simulink model "Demo_CarRealTime2D_cs"  (R2014b)
settings: Solver=ode5  SolverMode=SingleTasking  StartTime=0.0  StopTime=inf  FixedStep=1/1000  RelTol=1e-3
PreLoadFcn:
  | mbxruntime.callbacks.PreLoadFcn(bdroot);
  | check_NUTS_defined;
  | assignin('base',['model_closed_' bdroot],false);
  | addpath('../includes_AEBS');
PostLoadFcn:
  | mbxruntime.callbacks.PostLoadFcn(bdroot);
InitFcn:
  | mbxruntime.callbacks.InitFcn(bdroot);
StartFcn:
  | mbxruntime.callbacks.StartFcn(bdroot);
StopFcn:
  | mbxruntime.callbacks.StopFcn(bdroot);;
  | 
model workspace: external: MAT-File .\Demo_CarRealTime2D_cs_hws.mat (data not in the file)
undefined symbols (not defined in the file or in its folder): Driver_Demands, mbxruntime, tabledata, vicrt_initcallback, vicrt_initmexcallback, vicrt_simulationmanager, warningInitialVelocity, x0
undefined symbols (not defined in the file): Demo_CarRealTime2D_cs_007c1c37f387f47f, Demo_CarRealTime2D_cs_085a64a83ba38cec, Demo_CarRealTime2D_cs_0a7f542d3fc7ab9f, Demo_CarRealTime2D_cs_0d7c72cfaa56dff7, Demo_CarRealTime2D_cs_0de07b35068e3828, Demo_CarRealTime2D_cs_17f4d381375cce95, Demo_CarRealTime2D_cs_1db40a09b08215a9, Demo_CarRealTime2D_cs_2bfa3850c176687b, Demo_CarRealTime2D_cs_35a34f1ba6ce4a22, Demo_CarRealTime2D_cs_378cc77e08d643fb, Demo_CarRealTime2D_cs_409b5c3befba0000, Demo_CarRealTime2D_cs_42628ca5bb62d2f3, Demo_CarRealTime2D_cs_56554a2db408a7f8, Demo_CarRealTime2D_cs_59527455249d7429, Demo_CarRealTime2D_cs_5983ee1b8112afac, Demo_CarRealTime2D_cs_5b5ebcf3ed7bf8e6, Demo_CarRealTime2D_cs_63cbe7fbe16cd5d9, Demo_CarRealTime2D_cs_6e17b9adbf989abf, Demo_CarRealTime2D_cs_6f662a34e5d9a196, Demo_CarRealTime2D_cs_75c4ee8892821e19, Demo_CarRealTime2D_cs_7c64486355814be2, Demo_CarRealTime2D_cs_849809550a2230ef, Demo_CarRealTime2D_cs_87f899bcbe16d8f5, Demo_CarRealTime2D_cs_8e7b50dac25b68a2, Demo_CarRealTime2D_cs_94938e5260f139b3, Demo_CarRealTime2D_cs_983acc940698d1d1, Demo_CarRealTime2D_cs_9d554c72797f76fd, Demo_CarRealTime2D_cs_9d747ee2f15c057f, Demo_CarRealTime2D_cs_ad62a2084d31e898, Demo_CarRealTime2D_cs_b56c8c5f000d30f0, Demo_CarRealTime2D_cs_b95f1b7356e926cc, Demo_CarRealTime2D_cs_BMW_X5_1_Path_pathUniqueID, Demo_CarRealTime2D_cs_BMW_Z3_2_Dynamics_Empty_STATE_BMW_Z3_2_x0, Demo_CarRealTime2D_cs_BMW_Z3_2_Dynamics_Empty_STATE_BMW_Z3_2_y0, Demo_CarRealTime2D_cs_BMW_Z3_2_Dynamics_Empty_STATE_BMW_Z3_2_z0, Demo_CarRealTime2D_cs_BMW_Z3_Path_pathUniqueID, Demo_CarRealTime2D_cs_BMW_Z3_SpeedProfile_speedProfileUniqueID, Demo_CarRealTime2D_cs_c8847ab2e5633224, Demo_CarRealTime2D_cs_c9a0d701286b93fb, Demo_CarRealTime2D_cs_ce758cae7dd1b283, Demo_CarRealTime2D_cs_CrossingPedestrian_Path_pathUniqueID, Demo_CarRealTime2D_cs_CuttingInVehicle_Path_pathUniqueID, Demo_CarRealTime2D_cs_d901ab1c1d2e40bc, Demo_CarRealTime2D_cs_dff70430e5a00a86, Demo_CarRealTime2D_cs_ef038a4f619ad32e, Demo_CarRealTime2D_cs_Female_OverweightAni_1_Path_pathUniqueID, Demo_CarRealTime2D_cs_Ford_Fiesta_1_Path_pathUniqueID, Demo_CarRealTime2D_cs_Ford_FocusWagon_Path_pathUniqueID, Demo_CarRealTime2D_cs_Sphere_1_Dynamics_Empty_STATE_Sphere_1_x0, Demo_CarRealTime2D_cs_Sphere_1_Dynamics_Empty_STATE_Sphere_1_y0, Demo_CarRealTime2D_cs_Sphere_1_Dynamics_Empty_STATE_Sphere_1_z0, WheelL0, WheelL1, WheelR0, WheelR1
libraries: PreScanSimulinkLibrary x15, simulink x15, simulink_extras x15, PreScanUsefulBlocks x2, dspsigops x1
(part 16 of 17)

== system Demo_CarRealTime2D_cs/HostVehicle/PathFollower_Preview_1/LateralController/SteeringWheelAngle/FirstOrderDynamics ==
  In : Inport
  TimeConstant[s] : Inport  Port=2
  Reset : Inport  Port=3
  x0 : Inport  Port=4
  1|TimeConstant : Product  Inputs=*/  SaturateOnIntegerOverflow=on  InputSameDT=on  OutDataTypeStr=Inherit: Same as first input
  Discrete-Time Integrator : DiscreteIntegrator  ExternalReset=rising  InitialConditionSource=external  InitialCondition=x0  SampleTime=CSSampleTime
  IC : InitialCondition  Value=0
  Saturation : Saturate  UpperLimit=1e300  LowerLimit=0.001
  Sum : Sum  Inputs=-+|  SaturateOnIntegerOverflow=on  InputSameDT=on  OutDataTypeStr=Inherit: Same as first input
  Out : Outport
  wires:
  IC/1 -> Discrete-Time Integrator/3
  In/1 -> Sum/2
  x0/1 -> IC/1
  Reset/1 -> Discrete-Time Integrator/2
  1|TimeConstant/1 -> Discrete-Time Integrator/1
  Sum/1 -> 1|TimeConstant/1
  Saturation/1 -> 1|TimeConstant/2
  TimeConstant[s]/1 -> Saturation/1
  Discrete-Time Integrator/1 -> Out/1, Sum/1

== system Demo_CarRealTime2D_cs/HostVehicle/PathFollower_Preview_1/LateralController/SteeringWheelAngle/Sat_Total ==
  In : Inport
  Sat_Limit : Inport  Port=2
  Gain1 : Gain  Gain=-1  SaturateOnIntegerOverflow=on  OutDataTypeStr=Inherit: Same as input  ParamDataTypeStr=Inherit: Same as input
  RelOp_UL : RelationalOperator
  RelOp_UL1 : RelationalOperator  Operator=<=
  Sum : Sum  Inputs=++|  SaturateOnIntegerOverflow=on
  Switch : Switch  Threshold=0.5  SaturateOnIntegerOverflow=on
  Switch1 : Switch  Threshold=0.5  SaturateOnIntegerOverflow=on
  Sat_Total : Outport
  Sat_Info : Outport  Port=2
  wires:
  Sat_Limit/1 -> Gain1/1, Switch/1, RelOp_UL/2
  RelOp_UL/1 -> Switch/2, Sum/2
  Switch/1 -> RelOp_UL1/1, Switch1/3
  Gain1/1 -> RelOp_UL1/2, Switch1/1
  RelOp_UL1/1 -> Switch1/2, Sum/1
  In/1 -> Switch/3, RelOp_UL/1
  Switch1/1 -> Sat_Total/1
  Sum/1 -> Sat_Info/1

== system Demo_CarRealTime2D_cs/HostVehicle/PathFollower_Preview_1/LongitudinalController/If Desired Velocity ~= 0/PID_AWU ==
  e : Inport
  Derivative Gain : Gain  Gain=D  SaturateOnIntegerOverflow=on  OutDataTypeStr=Inherit: Same as input  ParamDataTypeStr=Inherit: Same as input
  Discrete-Time Integrator : DiscreteIntegrator  gainval=1  SampleTime=CSSampleTime  UpperSaturationLimit=100  LowerSaturationLimit=-100
  Filter : DiscreteIntegrator  gainval=1  SampleTime=CSSampleTime
  Integral Gain : Gain  Gain=I  SaturateOnIntegerOverflow=on  OutDataTypeStr=Inherit: Same as input  ParamDataTypeStr=Inherit: Same as input
  Integral Gain1 : Gain  Gain=LongCtrl_AWU  SaturateOnIntegerOverflow=on  OutDataTypeStr=Inherit: Same as input  ParamDataTypeStr=Inherit: Same as input
  Proportional Gain : Gain  Gain=P  SaturateOnIntegerOverflow=on  OutDataTypeStr=Inherit: Same as input  ParamDataTypeStr=Inherit: Same as input
  Saturation : Saturate  UpperLimit=100  LowerLimit=-100
  Sum : Sum  Inputs=+++  SaturateOnIntegerOverflow=on  InputSameDT=on  OutDataTypeStr=Inherit: Same as first input
  Sum1 : Sum  Inputs=|+-  SaturateOnIntegerOverflow=on  InputSameDT=on  OutDataTypeStr=Inherit: Same as first input
  Sum2 : Sum  Inputs=|++  SaturateOnIntegerOverflow=on  InputSameDT=on  OutDataTypeStr=Inherit: Same as first input
  Sum3 : Sum  Inputs=-+|  SaturateOnIntegerOverflow=on  InputSameDT=on  OutDataTypeStr=Inherit: Same as first input
  u : Outport  InitialOutput=0
  wires:
  Integral Gain1/1 -> Sum2/2
  Sum3/1 -> Integral Gain1/1
  Saturation/1 -> Sum3/2, u/1
  Sum2/1 -> Discrete-Time Integrator/1
  Sum1/1 -> Sum/3, Filter/1
  Filter/1 -> Sum1/2
  Derivative Gain/1 -> Sum1/1
  Sum/1 -> Sum3/1, Saturation/1
  e/1 -> Integral Gain/1, Proportional Gain/1, Derivative Gain/1
  Discrete-Time Integrator/1 -> Sum/2
  Proportional Gain/1 -> Sum/1
  Integral Gain/1 -> Sum2/1

== system Demo_CarRealTime2D_cs/HostVehicle/Vehicles Synchronization/Evaluate_Event_To_Trigger_CuttingVehicle/Evaluate Experiment Conditions /Compute Components ==
  R [m] : Inport
  Th [deg] : Inport  Port=2
  Degrees to Radians : simulink_extras/Transformations/Degrees to Radians
  Product1 : Product  RndMeth=Zero
  Product8 : Product  RndMeth=Zero
  Trigonometric Function1 : Trigonometry  Operator=cos
  Trigonometric Function3 : Trigonometry
  delta_x [m] : Outport
  delta_y [m] : Outport  Port=2
  wires:
  Th [deg]/1 -> Degrees to Radians/1
  Product1/1 -> delta_y [m]/1
  Trigonometric Function3/1 -> Product1/2
  Product8/1 -> delta_x [m]/1
  Trigonometric Function1/1 -> Product8/2
  R [m]/1 -> Product8/1, Product1/1
  Degrees to Radians/1 -> Trigonometric Function1/1, Trigonometric Function3/1

== system Demo_CarRealTime2D_cs/HostVehicle/Vehicles Synchronization/Evaluate_Event_To_Trigger_CuttingVehicle/Evaluate Experiment Conditions /Compute Relative Longitudional Velocity ==
  V_Det [m/s] : Inport
  HV_V [m/s] : Inport  Port=2
  Abs : Abs
  Sum : Sum  Inputs=|+-
  delta_V [m/s] : Outport
  wires:
  Abs/1 -> delta_V [m/s]/1
  Sum/1 -> Abs/1
  HV_V [m/s]/1 -> Sum/2
  V_Det [m/s]/1 -> Sum/1

== system Demo_CarRealTime2D_cs/HostVehicle/Vehicles Synchronization/Evaluate_Event_To_Trigger_CuttingVehicle/Evaluate Experiment Conditions /Compute Vehcile Position Bend Road ==
  R [m] : Inport
  Th [deg] : Inport  Port=2
  delta_x [m] : Inport  Port=3
  HV_V [m/s] : Inport  Port=4
  HV_YawRate [deg/s] : Inport  Port=5
  Action Port : ActionPort
  Compare To Constant : simulink/Logic and Bit Operations/Compare To Constant  relop=<  const=0  OutDataTypeStr=boolean
  Compare To Constant1 : simulink/Logic and Bit Operations/Compare To Constant  relop=>  const=0  OutDataTypeStr=boolean
  Compare To Constant2 : simulink/Logic and Bit Operations/Compare To Constant  relop=>  const=0  OutDataTypeStr=boolean
  Compare To Constant3 : simulink/Logic and Bit Operations/Compare To Constant  relop=<  const=0  OutDataTypeStr=boolean
  Dead Zone : DeadZone  LowerValue=-0.1  UpperValue=0.1  SaturateOnIntegerOverflow=on
  Dead Zone1 : DeadZone  LowerValue=-0.1  UpperValue=0.1  SaturateOnIntegerOverflow=on
  Scope : Scope
      settings: YMin=-2.75  YMax=0.25  SaveName=ScopeData2
  Sign : Signum
  Sign1 : Signum
  TV on same lane : Subsystem
  "TV_front " : Outport
  TV_rear : Outport  Port=2
  TV_left : Outport  Port=3
  TV_right : Outport  Port=4
  y_pos_traj : Outport  Port=5
  wires:
  Dead Zone1/1 -> Sign1/1
  Dead Zone/1 -> Sign/1
  Compare To Constant1/1 -> TV_right/1
  HV_YawRate [deg/s]/1 -> TV on same lane/4(HV_Yaw_rate_[deg/s])
  HV_V [m/s]/1 -> TV on same lane/3(HV_Velocity [m/s])
  Th [deg]/1 -> TV on same lane/2(Th_Sensor deg])
  R [m]/1 -> TV on same lane/1(Range_Sensor [m])
  delta_x [m]/1 -> Dead Zone/1
  Sign/1 -> Compare To Constant/1, Compare To Constant2/1
  Compare To Constant/1 -> TV_rear/1
  TV on same lane/1(y_pos_traj) -> y_pos_traj/1, Scope/1, Dead Zone1/1
  Sign1/1 -> Compare To Constant1/1, Compare To Constant3/1
  Compare To Constant2/1 -> "TV_front "/1
  Compare To Constant3/1 -> TV_left/1

== system Demo_CarRealTime2D_cs/HostVehicle/Vehicles Synchronization/Evaluate_Event_To_Trigger_CuttingVehicle/Evaluate Experiment Conditions /Compute Vehcile Position Sraight Road ==
  delta_x [m] : Inport
  delta_y [m] : Inport  Port=2
  Action Port : ActionPort
  Compare To Constant : simulink/Logic and Bit Operations/Compare To Constant  relop=<  const=0  OutDataTypeStr=boolean
  Compare To Constant1 : simulink/Logic and Bit Operations/Compare To Constant  relop=>  const=0  OutDataTypeStr=boolean
  Compare To Constant2 : simulink/Logic and Bit Operations/Compare To Constant  relop=>  const=0  OutDataTypeStr=boolean
  Compare To Constant3 : simulink/Logic and Bit Operations/Compare To Constant  relop=<  const=0  OutDataTypeStr=boolean
  Dead Zone : DeadZone  LowerValue=-0.1  UpperValue=0.1  SaturateOnIntegerOverflow=on
  Dead Zone1 : DeadZone  LowerValue=-0.1  UpperValue=0.1  SaturateOnIntegerOverflow=on
  Sign : Signum
  Sign1 : Signum
  "TV_front " : Outport
  TV_rear : Outport  Port=2
  TV_left : Outport  Port=3
  TV_right : Outport  Port=4
  wires:
  Dead Zone1/1 -> Sign1/1
  Dead Zone/1 -> Sign/1
  Compare To Constant3/1 -> TV_left/1
  Compare To Constant2/1 -> "TV_front "/1
  Compare To Constant1/1 -> TV_right/1
  Sign1/1 -> Compare To Constant3/1, Compare To Constant1/1
  delta_y [m]/1 -> Dead Zone1/1
  Compare To Constant/1 -> TV_rear/1
  Sign/1 -> Compare To Constant2/1, Compare To Constant/1
  delta_x [m]/1 -> Dead Zone/1

== system Demo_CarRealTime2D_cs/HostVehicle/Vehicles Synchronization/Evaluate_Event_To_Trigger_CuttingVehicle/Evaluate Experiment Conditions /Straight or Curved Road Scenario ==
  note: === Switching block ===
      |
      |  - determines if the HV is moving on a straight road or on a bend raod,
      |  - based on the actual value of the yaw rate of the HV.
  EGO_Yaw_rate_[deg/s] : Inport
  1deg_per_s : Constant
  Abs : Abs
  Bend_Road [2] : Constant  Value=2
  Relational Operator : RelationalOperator  Operator=<  OutDataTypeStr=boolean
  Straight_Road [1] : Constant
  Switch : Switch  Criteria=u2 ~= 0  Threshold=0.5
  Sraight[1] / Bend[2] : Outport
  wires:
  Bend_Road [2]/1 -> Switch/3
  Straight_Road [1]/1 -> Switch/1
  Abs/1 -> Relational Operator/1
  Switch/1 -> Sraight[1] / Bend[2]/1
  Relational Operator/1 -> Switch/2
  1deg_per_s/1 -> Relational Operator/2
  EGO_Yaw_rate_[deg/s]/1 -> Abs/1

== system Demo_CarRealTime2D_cs/CuttingInVehicle/Trajectories1/Traj2State1/Traj2State2/Traj2MuxState_Ext/demux ==
  traj : Inport
  Demux : Demux  Outputs=18
  x : Outport
  y : Outport  Port=2
  z : Outport  Port=3
  velx : Outport  Port=4
  vely : Outport  Port=5
  velz : Outport  Port=6
  R : Outport  Port=7
  P : Outport  Port=8
  Y : Outport  Port=9
  velR : Outport  Port=10
  velP : Outport  Port=11
  velY : Outport  Port=12
  accx : Outport  Port=13
  accy : Outport  Port=14
  accz : Outport  Port=15
  accR : Outport  Port=16
  accP : Outport  Port=17
  accY : Outport  Port=18
  wires:
  Demux/1 -> x/1
  Demux/2 -> y/1
  Demux/3 -> z/1
  Demux/4 -> R/1
  traj/1 -> Demux/1
  Demux/5 -> P/1
  Demux/6 -> Y/1
  Demux/7 -> velx/1
  Demux/8 -> vely/1
  Demux/9 -> velz/1
  Demux/10 -> velR/1
  Demux/11 -> velP/1
  Demux/12 -> velY/1
  Demux/13 -> accx/1
  Demux/14 -> accy/1
  Demux/15 -> accz/1
  Demux/16 -> accR/1
  Demux/17 -> accP/1
  Demux/18 -> accY/1

== system Demo_CarRealTime2D_cs/HostVehicle/Dynamics_UserSpecified/VI-CarRealTime/Input_Bus/Inputs/Aerodynamic ==
  BCAerodynamic : BusCreator  Inputs=12
  fx_center_def_val : Constant  Value=0
  fx_front_def_val : Constant  Value=0
  fx_rear_def_val : Constant  Value=0
  fy_center_def_val : Constant  Value=0
  fy_front_def_val : Constant  Value=0
  fy_rear_def_val : Constant  Value=0
  fz_center_def_val : Constant  Value=0
  fz_front_def_val : Constant  Value=0
  fz_rear_def_val : Constant  Value=0
  mx_def_val : Constant  Value=0
  my_def_val : Constant  Value=0
  mz_def_val : Constant  Value=0
  Aerodynamic : Outport
  wires:
  mz_def_val/1 -> BCAerodynamic/12  "mz"
  my_def_val/1 -> BCAerodynamic/11  "my"
  mx_def_val/1 -> BCAerodynamic/10  "mx"
  fz_center_def_val/1 -> BCAerodynamic/9  "fz_center"
  fy_center_def_val/1 -> BCAerodynamic/8  "fy_center"
  fx_center_def_val/1 -> BCAerodynamic/7  "fx_center"
  fz_rear_def_val/1 -> BCAerodynamic/6  "fz_rear"
  fy_rear_def_val/1 -> BCAerodynamic/5  "fy_rear"
  fx_rear_def_val/1 -> BCAerodynamic/4  "fx_rear"
  fz_front_def_val/1 -> BCAerodynamic/3  "fz_front"
  fy_front_def_val/1 -> BCAerodynamic/2  "fy_front"
  fx_front_def_val/1 -> BCAerodynamic/1  "fx_front"
  BCAerodynamic/1 -> Aerodynamic/1  "Aerodynamic"

== system Demo_CarRealTime2D_cs/HostVehicle/Dynamics_UserSpecified/VI-CarRealTime/Input_Bus/Inputs/Antiroll_Bar ==
  BCAntiroll_Bar : BusCreator  Inputs=2
  activity_flag : Subsystem
  force : Subsystem
  Antiroll_Bar : Outport
  wires:
  force/1(force) -> BCAntiroll_Bar/2  "force"
  activity_flag/1(activity_flag) -> BCAntiroll_Bar/1  "activity_flag"
  BCAntiroll_Bar/1 -> Antiroll_Bar/1  "Antiroll_Bar"

== system Demo_CarRealTime2D_cs/HostVehicle/Dynamics_UserSpecified/VI-CarRealTime/Input_Bus/Inputs/Auxiliary_vertical ==
  BCAuxiliary_vertical : BusCreator  Inputs=2
  activity_flag : Subsystem
  force : Subsystem
  Auxiliary_vertical : Outport
  wires:
  activity_flag/1(activity_flag) -> BCAuxiliary_vertical/2  "activity_flag"
  force/1(force) -> BCAuxiliary_vertical/1  "force"
  BCAuxiliary_vertical/1 -> Auxiliary_vertical/1  "Auxiliary_vertical"

== system Demo_CarRealTime2D_cs/HostVehicle/Dynamics_UserSpecified/VI-CarRealTime/Input_Bus/Inputs/Brake_System ==
  BCBrake_System : BusCreator  Inputs=5
  brk_mmag_sign : Subsystem
  brk_mmag_unsign : Subsystem
  brk_mu : Subsystem
  brk_pres : Subsystem
  brk_pres_gain : Subsystem
  Brake_System : Outport
  wires:
  brk_mu/1(brk_mu) -> BCBrake_System/5  "brk_mu"
  brk_pres_gain/1(brk_pres_gain) -> BCBrake_System/4  "brk_pres_gain"
  brk_pres/1(brk_pres) -> BCBrake_System/3  "brk_pres"
  brk_mmag_unsign/1(brk_mmag_unsign) -> BCBrake_System/2  "brk_mmag_unsign"
  brk_mmag_sign/1(brk_mmag_sign) -> BCBrake_System/1  "brk_mmag_sign"
  BCBrake_System/1 -> Brake_System/1  "Brake_System"

== system Demo_CarRealTime2D_cs/HostVehicle/Dynamics_UserSpecified/VI-CarRealTime/Input_Bus/Inputs/Brake_System_General ==
  BCBrake_System_General : BusCreator  Inputs=2
  brk_bias_front_def_val : Constant  Value=0
  brk_mast_cyl_pres_def_val : Constant  Value=0
  Brake_System_General : Outport
  wires:
  brk_bias_front_def_val/1 -> BCBrake_System_General/2  "brk_bias_front"
  brk_mast_cyl_pres_def_val/1 -> BCBrake_System_General/1  "brk_mast_cyl_pres"
  BCBrake_System_General/1 -> Brake_System_General/1  "Brake_System_General"

== system Demo_CarRealTime2D_cs/HostVehicle/Dynamics_UserSpecified/VI-CarRealTime/Input_Bus/Inputs/Clutch ==
  BCClutch : BusCreator  Inputs=2
  clutch_slip_angle_def_val : Constant  Value=0
  clutch_trq_def_val : Constant  Value=0
  Clutch : Outport
  wires:
  clutch_slip_angle_def_val/1 -> BCClutch/2  "clutch_slip_angle"
  clutch_trq_def_val/1 -> BCClutch/1  "clutch_trq"
  BCClutch/1 -> Clutch/1  "Clutch"

== system Demo_CarRealTime2D_cs/HostVehicle/Dynamics_UserSpecified/VI-CarRealTime/Input_Bus/Inputs/Driver_Demands ==
  BCDriver_Demands : BusCreator  Inputs=12
  brake_def_val : Constant  Value=0
  clutch_def_val : Constant  Value=0
  gear_def_val : Constant  Value=0
  rack_displacement_def_val : Constant  Value=0
  str_swa_def_val : Constant  Value=0
  throttle_def_val : Constant  Value=0
  user_input_braking_def_val : Constant  Value=0
  user_input_clutch_def_val : Constant  Value=0
  user_input_gear_def_val : Constant  Value=0
  user_input_steering_def_val : Constant  Value=0
  user_input_throttle_def_val : Constant  Value=0
  user_maneuver_ID_def_val : Constant  Value=0
  Driver_Demands : Outport
  wires:
  user_input_clutch_def_val/1 -> BCDriver_Demands/12  "user_input_clutch"
  user_input_gear_def_val/1 -> BCDriver_Demands/11  "user_input_gear"
  user_input_braking_def_val/1 -> BCDriver_Demands/10  "user_input_braking"
  user_input_throttle_def_val/1 -> BCDriver_Demands/9  "user_input_throttle"
  user_input_steering_def_val/1 -> BCDriver_Demands/8  "user_input_steering"
  user_maneuver_ID_def_val/1 -> BCDriver_Demands/7  "user_maneuver_ID"
  brake_def_val/1 -> BCDriver_Demands/6  "brake"
  clutch_def_val/1 -> BCDriver_Demands/5  "clutch"
  gear_def_val/1 -> BCDriver_Demands/4  "gear"
  throttle_def_val/1 -> BCDriver_Demands/3  "throttle"
  rack_displacement_def_val/1 -> BCDriver_Demands/2  "rack_displacement"
  str_swa_def_val/1 -> BCDriver_Demands/1  "str_swa"
  BCDriver_Demands/1 -> Driver_Demands/1  "Driver_Demands"

== system Demo_CarRealTime2D_cs/HostVehicle/Dynamics_UserSpecified/VI-CarRealTime/Input_Bus/Inputs/Engine ==
  BCEngine : BusCreator  Inputs=5
  engine_max_trq_def_val : Constant  Value=0
  engine_min_trq_def_val : Constant  Value=0
  engine_omega_def_val : Constant  Value=0
  engine_trq_def_val : Constant  Value=0
  non_termic_engine_trq_def_val : Constant  Value=0
  Engine : Outport
  wires:
  non_termic_engine_trq_def_val/1 -> BCEngine/5  "non_termic_engine_trq"
  engine_trq_def_val/1 -> BCEngine/4  "engine_trq"
  engine_min_trq_def_val/1 -> BCEngine/3  "engine_min_trq"
  engine_max_trq_def_val/1 -> BCEngine/2  "engine_max_trq"
  engine_omega_def_val/1 -> BCEngine/1  "engine_omega"
  BCEngine/1 -> Engine/1  "Engine"

== system Demo_CarRealTime2D_cs/HostVehicle/Dynamics_UserSpecified/VI-CarRealTime/Input_Bus/Inputs/Ext_Body ==
  BCExt_Body : BusCreator  Inputs=2
  force : Subsystem
  moment : Subsystem
  Ext_Body : Outport
  wires:
  moment/1(moment) -> BCExt_Body/2  "moment"
  force/1(force) -> BCExt_Body/1  "force"
  BCExt_Body/1 -> Ext_Body/1  "Ext_Body"

== system Demo_CarRealTime2D_cs/HostVehicle/Dynamics_UserSpecified/VI-CarRealTime/Input_Bus/Inputs/Ext_Ground ==
  BCExt_Ground : BusCreator  Inputs=2
  force : Subsystem
  moment : Subsystem
  Ext_Ground : Outport
  wires:
  moment/1(moment) -> BCExt_Ground/2  "moment"
  force/1(force) -> BCExt_Ground/1  "force"
  BCExt_Ground/1 -> Ext_Ground/1  "Ext_Ground"

== system Demo_CarRealTime2D_cs/HostVehicle/Dynamics_UserSpecified/VI-CarRealTime/Input_Bus/Inputs/Ext_Tracking ==
  BCExt_Tracking : BusCreator  Inputs=2
  force : Subsystem
  moment : Subsystem
  Ext_Tracking : Outport
  wires:
  moment/1(moment) -> BCExt_Tracking/2  "moment"
  force/1(force) -> BCExt_Tracking/1  "force"
  BCExt_Tracking/1 -> Ext_Tracking/1  "Ext_Tracking"

== system Demo_CarRealTime2D_cs/HostVehicle/Dynamics_UserSpecified/VI-CarRealTime/Input_Bus/Inputs/Friction ==
  BCFriction : BusCreator  Inputs=1
  tire_mu : Subsystem
  Friction : Outport
  wires:
  tire_mu/1(tire_mu) -> BCFriction/1  "tire_mu"
  BCFriction/1 -> Friction/1  "Friction"

== system Demo_CarRealTime2D_cs/HostVehicle/Dynamics_UserSpecified/VI-CarRealTime/Input_Bus/Inputs/GearBox ==
  BCGearBox : BusCreator  Inputs=1
  transmission_ratio_def_val : Constant  Value=0
  GearBox : Outport
  wires:
  transmission_ratio_def_val/1 -> BCGearBox/1  "transmission_ratio"
  BCGearBox/1 -> GearBox/1  "GearBox"

== system Demo_CarRealTime2D_cs/HostVehicle/Dynamics_UserSpecified/VI-CarRealTime/Input_Bus/Inputs/Hook ==
  BCHook : BusCreator  Inputs=6
  Fx : Subsystem
  Fy : Subsystem
  Fz : Subsystem
  Mx : Subsystem
  My : Subsystem
  Mz : Subsystem
  Hook : Outport
  wires:
  Mz/1(Mz) -> BCHook/6  "Mz"
  My/1(My) -> BCHook/5  "My"
  Mx/1(Mx) -> BCHook/4  "Mx"
  Fz/1(Fz) -> BCHook/3  "Fz"
  Fy/1(Fy) -> BCHook/2  "Fy"
  Fx/1(Fx) -> BCHook/1  "Fx"
  BCHook/1 -> Hook/1  "Hook"

== system Demo_CarRealTime2D_cs/HostVehicle/Dynamics_UserSpecified/VI-CarRealTime/Input_Bus/Inputs/Irregularity ==
  BCIrregularity : BusCreator  Inputs=1
  road : Subsystem
  Irregularity : Outport
  wires:
  road/1(road) -> BCIrregularity/1  "road"
  BCIrregularity/1 -> Irregularity/1  "Irregularity"

== system Demo_CarRealTime2D_cs/HostVehicle/Dynamics_UserSpecified/VI-CarRealTime/Input_Bus/Inputs/Main_Bumpstop ==
  BCMain_Bumpstop : BusCreator  Inputs=2
  activity_flag : Subsystem
  force : Subsystem
  Main_Bumpstop : Outport
  wires:
  activity_flag/1(activity_flag) -> BCMain_Bumpstop/2  "activity_flag"
  force/1(force) -> BCMain_Bumpstop/1  "force"
  BCMain_Bumpstop/1 -> Main_Bumpstop/1  "Main_Bumpstop"

== system Demo_CarRealTime2D_cs/HostVehicle/Dynamics_UserSpecified/VI-CarRealTime/Input_Bus/Inputs/Main_Damper ==
  BCMain_Damper : BusCreator  Inputs=2
  activity_flag : Subsystem
  force : Subsystem
  Main_Damper : Outport
  wires:
  activity_flag/1(activity_flag) -> BCMain_Damper/2  "activity_flag"
  force/1(force) -> BCMain_Damper/1  "force"
  BCMain_Damper/1 -> Main_Damper/1  "Main_Damper"

== system Demo_CarRealTime2D_cs/HostVehicle/Dynamics_UserSpecified/VI-CarRealTime/Input_Bus/Inputs/Main_Reboundstop ==
  BCMain_Reboundstop : BusCreator  Inputs=2
  activity_flag : Subsystem
  force : Subsystem
  Main_Reboundstop : Outport
  wires:
  activity_flag/1(activity_flag) -> BCMain_Reboundstop/2  "activity_flag"
  force/1(force) -> BCMain_Reboundstop/1  "force"
  BCMain_Reboundstop/1 -> Main_Reboundstop/1  "Main_Reboundstop"

== system Demo_CarRealTime2D_cs/HostVehicle/Dynamics_UserSpecified/VI-CarRealTime/Input_Bus/Inputs/Main_Spring ==
  BCMain_Spring : BusCreator  Inputs=2
  activity_flag : Subsystem
  force : Subsystem
  Main_Spring : Outport
  wires:
  activity_flag/1(activity_flag) -> BCMain_Spring/2  "activity_flag"
  force/1(force) -> BCMain_Spring/1  "force"
  BCMain_Spring/1 -> Main_Spring/1  "Main_Spring"

== system Demo_CarRealTime2D_cs/HostVehicle/Dynamics_UserSpecified/VI-CarRealTime/Input_Bus/Inputs/Mono_Element ==
  BCMono_Element : BusCreator  Inputs=14
  Bumpstop_Damper : Subsystem
  Bumpstop_Damper_activity_flag : Subsystem
  Bumpstop_Spring : Subsystem
  Bumpstop_Spring_activity_flag : Subsystem
  Damper : Subsystem
  Damper_activity_flag : Subsystem
  Inerter : Subsystem
  Inerter_activity_flag : Subsystem
  Reboundstop_Damper : Subsystem
  Reboundstop_Damper_activity_flag : Subsystem
  Reboundstop_Spring : Subsystem
  Reboundstop_Spring_activity_flag : Subsystem
  Spring : Subsystem
  Spring_activity_flag : Subsystem
  Mono_Element : Outport
  wires:
  Reboundstop_Damper_activity_flag/1(Reboundstop_Damper_activity_flag) -> BCMono_Element/14  "Reboundstop_Damper_activity_flag"
  Reboundstop_Damper/1(Reboundstop_Damper) -> BCMono_Element/13  "Reboundstop_Damper"
  Bumpstop_Damper_activity_flag/1(Bumpstop_Damper_activity_flag) -> BCMono_Element/12  "Bumpstop_Damper_activity_flag"
  Bumpstop_Damper/1(Bumpstop_Damper) -> BCMono_Element/11  "Bumpstop_Damper"
  Reboundstop_Spring_activity_flag/1(Reboundstop_Spring_activity_flag) -> BCMono_Element/10  "Reboundstop_Spring_activity_flag"
  Reboundstop_Spring/1(Reboundstop_Spring) -> BCMono_Element/9  "Reboundstop_Spring"
  Bumpstop_Spring_activity_flag/1(Bumpstop_Spring_activity_flag) -> BCMono_Element/8  "Bumpstop_Spring_activity_flag"
  Bumpstop_Spring/1(Bumpstop_Spring) -> BCMono_Element/7  "Bumpstop_Spring"
  Spring_activity_flag/1(Spring_activity_flag) -> BCMono_Element/6  "Spring_activity_flag"
  Spring/1(Spring) -> BCMono_Element/5  "Spring"
  Inerter_activity_flag/1(Inerter_activity_flag) -> BCMono_Element/4  "Inerter_activity_flag"
  Inerter/1(Inerter) -> BCMono_Element/3  "Inerter"
  Damper_activity_flag/1(Damper_activity_flag) -> BCMono_Element/2  "Damper_activity_flag"
  Damper/1(Damper) -> BCMono_Element/1  "Damper"
  BCMono_Element/1 -> Mono_Element/1  "Mono_Element"

== system Demo_CarRealTime2D_cs/HostVehicle/Dynamics_UserSpecified/VI-CarRealTime/Input_Bus/Inputs/Rear_Steering_Actuator_disp ==
  BCRear_Steering_Actuator_disp : BusCreator  Inputs=1
  str_swa : Subsystem
  Rear_Steering_Actuator_disp : Outport
  wires:
  str_swa/1(str_swa) -> BCRear_Steering_Actuator_disp/1  "str_swa"
  BCRear_Steering_Actuator_disp/1 -> Rear_Steering_Actuator_disp/1  "Rear_Steering_Actuator_disp"

== system Demo_CarRealTime2D_cs/HostVehicle/Dynamics_UserSpecified/VI-CarRealTime/Input_Bus/Inputs/Steering ==
  BCSteering : BusCreator  Inputs=1
  steer_at_spindle : Subsystem
  Steering : Outport
  wires:
  steer_at_spindle/1(steer_at_spindle) -> BCSteering/1  "steer_at_spindle"
  BCSteering/1 -> Steering/1  "Steering"

== system Demo_CarRealTime2D_cs/HostVehicle/Dynamics_UserSpecified/VI-CarRealTime/Input_Bus/Inputs/Subsystem_Activation ==
  BCSubsystem_Activation : BusCreator  Inputs=12
  Internal_Aero_Activity_def_val : Constant
  Internal_Brake_System_Activity : Subsystem
  Internal_Clutch_Activity_def_val : Constant
  Internal_Engine_Activity_def_val : Constant
  Internal_Gearbox_Activity_def_val : Constant
  Internal_Steering_Column_Activity_def_val : Constant
  Tire_Force_x : Subsystem
  Tire_Force_y : Subsystem
  Tire_Force_z : Subsystem
  Tire_Moment_x : Subsystem
  Tire_Moment_y : Subsystem
  Tire_Moment_z : Subsystem
  Subsystem_Activation : Outport
  wires:
  Tire_Moment_z/1(Tire_Moment_z) -> BCSubsystem_Activation/12  "Tire_Moment_z"
  Tire_Moment_y/1(Tire_Moment_y) -> BCSubsystem_Activation/11  "Tire_Moment_y"
  Tire_Moment_x/1(Tire_Moment_x) -> BCSubsystem_Activation/10  "Tire_Moment_x"
  Tire_Force_z/1(Tire_Force_z) -> BCSubsystem_Activation/9  "Tire_Force_z"
  Tire_Force_y/1(Tire_Force_y) -> BCSubsystem_Activation/8  "Tire_Force_y"
  Tire_Force_x/1(Tire_Force_x) -> BCSubsystem_Activation/7  "Tire_Force_x"
  Internal_Aero_Activity_def_val/1 -> BCSubsystem_Activation/6  "Internal_Aero_Activity"
  Internal_Gearbox_Activity_def_val/1 -> BCSubsystem_Activation/5  "Internal_Gearbox_Activity"
  Internal_Engine_Activity_def_val/1 -> BCSubsystem_Activation/4  "Internal_Engine_Activity"
  Internal_Clutch_Activity_def_val/1 -> BCSubsystem_Activation/3  "Internal_Clutch_Activity"
  Internal_Brake_System_Activity/1(Internal_Brake_System_Activity) -> BCSubsystem_Activation/2  "Internal_Brake_System_Activity"
  Internal_Steering_Column_Activity_def_val/1 -> BCSubsystem_Activation/1  "Internal_Steering_Column_Activity"
  BCSubsystem_Activation/1 -> Subsystem_Activation/1  "Subsystem_Activation"

== system Demo_CarRealTime2D_cs/HostVehicle/Dynamics_UserSpecified/VI-CarRealTime/Input_Bus/Inputs/Third_Element ==
  BCThird_Element : BusCreator
  Damper_activity_flag : Subsystem
  Damper_force : Subsystem
  Spring : Subsystem
  Spring_activity_flag : Subsystem
  Third_Element : Outport
  wires:
  Spring_activity_flag/1(Spring_activity_flag) -> BCThird_Element/4  "Spring_activity_flag"
  Spring/1(Spring) -> BCThird_Element/3  "Spring"
  Damper_activity_flag/1(Damper_activity_flag) -> BCThird_Element/2  "Damper_activity_flag"
  Damper_force/1(Damper_force) -> BCThird_Element/1  "Damper_force"
  BCThird_Element/1 -> Third_Element/1  "Third_Element"

== system Demo_CarRealTime2D_cs/HostVehicle/Dynamics_UserSpecified/VI-CarRealTime/Input_Bus/Inputs/Tire_Force ==
  BCTire_Force : BusCreator  Inputs=3
  Fx : Subsystem
  Fy : Subsystem
  Fz : Subsystem
  Tire_Force : Outport
  wires:
  Fz/1(Fz) -> BCTire_Force/3  "Fz"
  Fy/1(Fy) -> BCTire_Force/2  "Fy"
  Fx/1(Fx) -> BCTire_Force/1  "Fx"
  BCTire_Force/1 -> Tire_Force/1  "Tire_Force"

== system Demo_CarRealTime2D_cs/HostVehicle/Dynamics_UserSpecified/VI-CarRealTime/Input_Bus/Inputs/Tire_Moment ==
  BCTire_Moment : BusCreator  Inputs=3
  Mx : Subsystem
  My : Subsystem
  Mz : Subsystem
  Tire_Moment : Outport
  wires:
  Mz/1(Mz) -> BCTire_Moment/3  "Mz"
  My/1(My) -> BCTire_Moment/2  "My"
  Mx/1(Mx) -> BCTire_Moment/1  "Mx"
  BCTire_Moment/1 -> Tire_Moment/1  "Tire_Moment"

== system Demo_CarRealTime2D_cs/HostVehicle/Dynamics_UserSpecified/VI-CarRealTime/Input_Bus/Inputs/Wheel_driving ==
  BCWheel_driving : BusCreator  Inputs=1
  moment : Subsystem
  Wheel_driving : Outport
  wires:
  moment/1(moment) -> BCWheel_driving/1  "moment"
  BCWheel_driving/1 -> Wheel_driving/1  "Wheel_driving"

== system Demo_CarRealTime2D_cs/HostVehicle/Vehicles Synchronization/Evaluate_Event_To_Trigger_CuttingVehicle/Evaluate Experiment Conditions /Compute Vehcile Position Bend Road/TV on same lane ==
  note: === TIS1 Objects On Lane block ===
      |
      |  - decides which objects are on the same lane as the EGO car,
      |     when the EGO car drives through the bend road.
  Range_Sensor [m] : Inport
  Th_Sensor deg] : Inport  Port=2
  HV_Velocity [m/s] : Inport  Port=3
  HV_Yaw_rate_[deg/s] : Inport  Port=4
  Abs : Abs
  Add4 : Sum  Inputs=++-
  Add6 : Sum  Inputs=+-
  Degrees to Radians : simulink_extras/Transformations/Degrees to Radians
  Degrees to Radians1 : simulink_extras/Transformations/Degrees to Radians
  Divide : Product  Inputs=*/
  Gain : Gain  Gain=2
  HV_Yaw_rate_[deg/s]1 : InportShadow  Port=4
  Product7 : Product  RndMeth=Zero
  Product8 : Product  RndMeth=Zero
  Product9 : Product  Inputs=3  RndMeth=Zero
  Sqrt1 : Math  Operator=sqrt  SaturateOnIntegerOverflow=on
  Switch4 : Switch  Criteria=u2 > Threshold
  Trigonometric Function3 : Trigonometry
  Unary Minus1 : UnaryMinus
  y_pos_traj : Outport
  wires:
  Degrees to Radians1/1 -> Divide/2
  Th_Sensor deg]/1 -> Switch4/3, Unary Minus1/1
  Unary Minus1/1 -> Switch4/1
  Degrees to Radians/1 -> Trigonometric Function3/1
  HV_Yaw_rate_[deg/s]1/1 -> Switch4/2
  Abs/1 -> Degrees to Radians1/1
  Range_Sensor [m]/1 -> Product9/2, Product7/2, Product7/1
  Switch4/1 -> Degrees to Radians/1
  Add6/1 -> y_pos_traj/1
  Sqrt1/1 -> Add6/1
  Add4/1 -> Sqrt1/1
  Trigonometric Function3/1 -> Product9/3
  Product9/1 -> Gain/1
  Gain/1 -> Add4/3
  Product7/1 -> Add4/2
  Product8/1 -> Add4/1
  Divide/1 -> Add6/2, Product9/1, Product8/2, Product8/1
  HV_Yaw_rate_[deg/s]/1 -> Abs/1
  HV_Velocity [m/s]/1 -> Divide/1

== system Demo_CarRealTime2D_cs/HostVehicle/Dynamics_UserSpecified/VI-CarRealTime/Input_Bus/Inputs/Antiroll_Bar/activity_flag ==
  BCactivity_flag : BusCreator  Inputs=2
  front_def_val : Constant
  rear_def_val : Constant
  activity_flag : Outport
  wires:
  rear_def_val/1 -> BCactivity_flag/2  "rear"
  front_def_val/1 -> BCactivity_flag/1  "front"
  BCactivity_flag/1 -> activity_flag/1  "activity_flag"

== system Demo_CarRealTime2D_cs/HostVehicle/Dynamics_UserSpecified/VI-CarRealTime/Input_Bus/Inputs/Antiroll_Bar/force ==
  BCforce : BusCreator  Inputs=2
  front_def_val : Constant  Value=0
  rear_def_val : Constant  Value=0
  force : Outport
  wires:
  rear_def_val/1 -> BCforce/2  "rear"
  front_def_val/1 -> BCforce/1  "front"
  BCforce/1 -> force/1  "force"

== system Demo_CarRealTime2D_cs/HostVehicle/Dynamics_UserSpecified/VI-CarRealTime/Input_Bus/Inputs/Auxiliary_vertical/activity_flag ==
  BCactivity_flag : BusCreator
  L1_def_val : Constant
  L2_def_val : Constant
  R1_def_val : Constant
  R2_def_val : Constant
  activity_flag : Outport
  wires:
  R2_def_val/1 -> BCactivity_flag/4  "R2"
  R1_def_val/1 -> BCactivity_flag/3  "R1"
  L2_def_val/1 -> BCactivity_flag/2  "L2"
  L1_def_val/1 -> BCactivity_flag/1  "L1"
  BCactivity_flag/1 -> activity_flag/1  "activity_flag"

== system Demo_CarRealTime2D_cs/HostVehicle/Dynamics_UserSpecified/VI-CarRealTime/Input_Bus/Inputs/Auxiliary_vertical/force ==
  BCforce : BusCreator
  L1_def_val : Constant  Value=0
  L2_def_val : Constant  Value=0
  R1_def_val : Constant  Value=0
  R2_def_val : Constant  Value=0
  force : Outport
  wires:
  R2_def_val/1 -> BCforce/4  "R2"
  R1_def_val/1 -> BCforce/3  "R1"
  L2_def_val/1 -> BCforce/2  "L2"
  L1_def_val/1 -> BCforce/1  "L1"
  BCforce/1 -> force/1  "force"

== system Demo_CarRealTime2D_cs/HostVehicle/Dynamics_UserSpecified/VI-CarRealTime/Input_Bus/Inputs/Brake_System/brk_mmag_sign ==
  BCbrk_mmag_sign : BusCreator
  L1_def_val : Constant  Value=0
  L2_def_val : Constant  Value=0
  R1_def_val : Constant  Value=0
  R2_def_val : Constant  Value=0
  brk_mmag_sign : Outport
  wires:
  R2_def_val/1 -> BCbrk_mmag_sign/4  "R2"
  R1_def_val/1 -> BCbrk_mmag_sign/3  "R1"
  L2_def_val/1 -> BCbrk_mmag_sign/2  "L2"
  L1_def_val/1 -> BCbrk_mmag_sign/1  "L1"
  BCbrk_mmag_sign/1 -> brk_mmag_sign/1  "brk_mmag_sign"

== system Demo_CarRealTime2D_cs/HostVehicle/Dynamics_UserSpecified/VI-CarRealTime/Input_Bus/Inputs/Brake_System/brk_mmag_unsign ==
  BCbrk_mmag_unsign : BusCreator
  L1_def_val : Constant  Value=0
  L2_def_val : Constant  Value=0
  R1_def_val : Constant  Value=0
  R2_def_val : Constant  Value=0
  brk_mmag_unsign : Outport
  wires:
  R2_def_val/1 -> BCbrk_mmag_unsign/4  "R2"
  R1_def_val/1 -> BCbrk_mmag_unsign/3  "R1"
  L2_def_val/1 -> BCbrk_mmag_unsign/2  "L2"
  L1_def_val/1 -> BCbrk_mmag_unsign/1  "L1"
  BCbrk_mmag_unsign/1 -> brk_mmag_unsign/1  "brk_mmag_unsign"

== system Demo_CarRealTime2D_cs/HostVehicle/Dynamics_UserSpecified/VI-CarRealTime/Input_Bus/Inputs/Brake_System/brk_mu ==
  BCbrk_mu : BusCreator
  L1_def_val : Constant  Value=0
  L2_def_val : Constant  Value=0
  R1_def_val : Constant  Value=0
  R2_def_val : Constant  Value=0
  brk_mu : Outport
  wires:
  R2_def_val/1 -> BCbrk_mu/4  "R2"
  R1_def_val/1 -> BCbrk_mu/3  "R1"
  L2_def_val/1 -> BCbrk_mu/2  "L2"
  L1_def_val/1 -> BCbrk_mu/1  "L1"
  BCbrk_mu/1 -> brk_mu/1  "brk_mu"

== system Demo_CarRealTime2D_cs/HostVehicle/Dynamics_UserSpecified/VI-CarRealTime/Input_Bus/Inputs/Brake_System/brk_pres ==
  BCbrk_pres : BusCreator
  L1_def_val : Constant  Value=0
  L2_def_val : Constant  Value=0
  R1_def_val : Constant  Value=0
  R2_def_val : Constant  Value=0
  brk_pres : Outport
  wires:
  R2_def_val/1 -> BCbrk_pres/4  "R2"
  R1_def_val/1 -> BCbrk_pres/3  "R1"
  L2_def_val/1 -> BCbrk_pres/2  "L2"
  L1_def_val/1 -> BCbrk_pres/1  "L1"
  BCbrk_pres/1 -> brk_pres/1  "brk_pres"

== system Demo_CarRealTime2D_cs/HostVehicle/Dynamics_UserSpecified/VI-CarRealTime/Input_Bus/Inputs/Brake_System/brk_pres_gain ==
  BCbrk_pres_gain : BusCreator
  L1_def_val : Constant
  L2_def_val : Constant
  R1_def_val : Constant
  R2_def_val : Constant
  brk_pres_gain : Outport
  wires:
  R2_def_val/1 -> BCbrk_pres_gain/4  "R2"
  R1_def_val/1 -> BCbrk_pres_gain/3  "R1"
  L2_def_val/1 -> BCbrk_pres_gain/2  "L2"
  L1_def_val/1 -> BCbrk_pres_gain/1  "L1"
  BCbrk_pres_gain/1 -> brk_pres_gain/1  "brk_pres_gain"

== system Demo_CarRealTime2D_cs/HostVehicle/Dynamics_UserSpecified/VI-CarRealTime/Input_Bus/Inputs/Ext_Body/force ==
  BCforce : BusCreator  Inputs=3
  X_def_val : Constant  Value=0
  Y_def_val : Constant  Value=0
  Z_def_val : Constant  Value=0
  force : Outport
  wires:
  Z_def_val/1 -> BCforce/3  "Z"
  Y_def_val/1 -> BCforce/2  "Y"
  X_def_val/1 -> BCforce/1  "X"
  BCforce/1 -> force/1  "force"

== system Demo_CarRealTime2D_cs/HostVehicle/Dynamics_UserSpecified/VI-CarRealTime/Input_Bus/Inputs/Ext_Body/moment ==
  BCmoment : BusCreator  Inputs=3
  X_def_val : Constant  Value=0
  Y_def_val : Constant  Value=0
  Z_def_val : Constant  Value=0
  moment : Outport
  wires:
  Z_def_val/1 -> BCmoment/3  "Z"
  Y_def_val/1 -> BCmoment/2  "Y"
  X_def_val/1 -> BCmoment/1  "X"
  BCmoment/1 -> moment/1  "moment"

== system Demo_CarRealTime2D_cs/HostVehicle/Dynamics_UserSpecified/VI-CarRealTime/Input_Bus/Inputs/Ext_Ground/force ==
  BCforce : BusCreator  Inputs=3
  X_def_val : Constant  Value=0
  Y_def_val : Constant  Value=0
  Z_def_val : Constant  Value=0
  force : Outport
  wires:
  Z_def_val/1 -> BCforce/3  "Z"
  Y_def_val/1 -> BCforce/2  "Y"
  X_def_val/1 -> BCforce/1  "X"
  BCforce/1 -> force/1  "force"

== system Demo_CarRealTime2D_cs/HostVehicle/Dynamics_UserSpecified/VI-CarRealTime/Input_Bus/Inputs/Ext_Ground/moment ==
  BCmoment : BusCreator  Inputs=3
  X_def_val : Constant  Value=0
  Y_def_val : Constant  Value=0
  Z_def_val : Constant  Value=0
  moment : Outport
  wires:
  Z_def_val/1 -> BCmoment/3  "Z"
  Y_def_val/1 -> BCmoment/2  "Y"
  X_def_val/1 -> BCmoment/1  "X"
  BCmoment/1 -> moment/1  "moment"

== system Demo_CarRealTime2D_cs/HostVehicle/Dynamics_UserSpecified/VI-CarRealTime/Input_Bus/Inputs/Ext_Tracking/force ==
  BCforce : BusCreator  Inputs=2
  X_def_val : Constant  Value=0
  Y_def_val : Constant  Value=0
  force : Outport
  wires:
  Y_def_val/1 -> BCforce/2  "Y"
  X_def_val/1 -> BCforce/1  "X"
  BCforce/1 -> force/1  "force"

== system Demo_CarRealTime2D_cs/HostVehicle/Dynamics_UserSpecified/VI-CarRealTime/Input_Bus/Inputs/Ext_Tracking/moment ==
  BCmoment : BusCreator  Inputs=2
  X_def_val : Constant  Value=0
  Y_def_val : Constant  Value=0
  moment : Outport
  wires:
  Y_def_val/1 -> BCmoment/2  "Y"
  X_def_val/1 -> BCmoment/1  "X"
  BCmoment/1 -> moment/1  "moment"

== system Demo_CarRealTime2D_cs/HostVehicle/Dynamics_UserSpecified/VI-CarRealTime/Input_Bus/Inputs/Friction/tire_mu ==
  BCtire_mu : BusCreator
  L1_def_val : Constant  Value=0
  L2_def_val : Constant  Value=0
  R1_def_val : Constant  Value=0
  R2_def_val : Constant  Value=0
  tire_mu : Outport
  wires:
  R2_def_val/1 -> BCtire_mu/4  "R2"
  R1_def_val/1 -> BCtire_mu/3  "R1"
  L2_def_val/1 -> BCtire_mu/2  "L2"
  L1_def_val/1 -> BCtire_mu/1  "L1"
  BCtire_mu/1 -> tire_mu/1  "tire_mu"

== system Demo_CarRealTime2D_cs/HostVehicle/Dynamics_UserSpecified/VI-CarRealTime/Input_Bus/Inputs/Hook/Fx ==
  BCFx : BusCreator  Inputs=1
  rear_def_val : Constant  Value=0
  Fx : Outport
  wires:
  rear_def_val/1 -> BCFx/1  "rear"
  BCFx/1 -> Fx/1  "Fx"

== system Demo_CarRealTime2D_cs/HostVehicle/Dynamics_UserSpecified/VI-CarRealTime/Input_Bus/Inputs/Hook/Fy ==
  BCFy : BusCreator  Inputs=1
  rear_def_val : Constant  Value=0
  Fy : Outport
  wires:
  rear_def_val/1 -> BCFy/1  "rear"
  BCFy/1 -> Fy/1  "Fy"

== system Demo_CarRealTime2D_cs/HostVehicle/Dynamics_UserSpecified/VI-CarRealTime/Input_Bus/Inputs/Hook/Fz ==
  BCFz : BusCreator  Inputs=1
  rear_def_val : Constant  Value=0
  Fz : Outport
  wires:
  rear_def_val/1 -> BCFz/1  "rear"
  BCFz/1 -> Fz/1  "Fz"

== system Demo_CarRealTime2D_cs/HostVehicle/Dynamics_UserSpecified/VI-CarRealTime/Input_Bus/Inputs/Hook/Mx ==
  BCMx : BusCreator  Inputs=1
  rear_def_val : Constant  Value=0
  Mx : Outport
  wires:
  rear_def_val/1 -> BCMx/1  "rear"
  BCMx/1 -> Mx/1  "Mx"

== system Demo_CarRealTime2D_cs/HostVehicle/Dynamics_UserSpecified/VI-CarRealTime/Input_Bus/Inputs/Hook/My ==
  BCMy : BusCreator  Inputs=1
  rear_def_val : Constant  Value=0
  My : Outport
  wires:
  rear_def_val/1 -> BCMy/1  "rear"
  BCMy/1 -> My/1  "My"

== system Demo_CarRealTime2D_cs/HostVehicle/Dynamics_UserSpecified/VI-CarRealTime/Input_Bus/Inputs/Hook/Mz ==
  BCMz : BusCreator  Inputs=1
  rear_def_val : Constant  Value=0
  Mz : Outport
  wires:
  rear_def_val/1 -> BCMz/1  "rear"
  BCMz/1 -> Mz/1  "Mz"

== system Demo_CarRealTime2D_cs/HostVehicle/Dynamics_UserSpecified/VI-CarRealTime/Input_Bus/Inputs/Irregularity/road ==
  BCroad : BusCreator
  L1_def_val : Constant  Value=0
  L2_def_val : Constant  Value=0
  R1_def_val : Constant  Value=0
  R2_def_val : Constant  Value=0
  road : Outport
  wires:
  R2_def_val/1 -> BCroad/4  "R2"
  R1_def_val/1 -> BCroad/3  "R1"
  L2_def_val/1 -> BCroad/2  "L2"
  L1_def_val/1 -> BCroad/1  "L1"
  BCroad/1 -> road/1  "road"

== system Demo_CarRealTime2D_cs/HostVehicle/Dynamics_UserSpecified/VI-CarRealTime/Input_Bus/Inputs/Main_Bumpstop/activity_flag ==
  BCactivity_flag : BusCreator
  L1_def_val : Constant
  L2_def_val : Constant
  R1_def_val : Constant
  R2_def_val : Constant
  activity_flag : Outport
  wires:
  R2_def_val/1 -> BCactivity_flag/4  "R2"
  R1_def_val/1 -> BCactivity_flag/3  "R1"
  L2_def_val/1 -> BCactivity_flag/2  "L2"
  L1_def_val/1 -> BCactivity_flag/1  "L1"
  BCactivity_flag/1 -> activity_flag/1  "activity_flag"

== system Demo_CarRealTime2D_cs/HostVehicle/Dynamics_UserSpecified/VI-CarRealTime/Input_Bus/Inputs/Main_Bumpstop/force ==
  BCforce : BusCreator
  L1_def_val : Constant  Value=0
  L2_def_val : Constant  Value=0
  R1_def_val : Constant  Value=0
  R2_def_val : Constant  Value=0
  force : Outport
  wires:
  R2_def_val/1 -> BCforce/4  "R2"
  R1_def_val/1 -> BCforce/3  "R1"
  L2_def_val/1 -> BCforce/2  "L2"
  L1_def_val/1 -> BCforce/1  "L1"
  BCforce/1 -> force/1  "force"

== system Demo_CarRealTime2D_cs/HostVehicle/Dynamics_UserSpecified/VI-CarRealTime/Input_Bus/Inputs/Main_Damper/activity_flag ==
  BCactivity_flag : BusCreator
  L1_def_val : Constant
  L2_def_val : Constant
  R1_def_val : Constant
  R2_def_val : Constant
  activity_flag : Outport
  wires:
  R2_def_val/1 -> BCactivity_flag/4  "R2"
  R1_def_val/1 -> BCactivity_flag/3  "R1"
  L2_def_val/1 -> BCactivity_flag/2  "L2"
  L1_def_val/1 -> BCactivity_flag/1  "L1"
  BCactivity_flag/1 -> activity_flag/1  "activity_flag"

== system Demo_CarRealTime2D_cs/HostVehicle/Dynamics_UserSpecified/VI-CarRealTime/Input_Bus/Inputs/Main_Damper/force ==
  BCforce : BusCreator
  L1_def_val : Constant  Value=0
  L2_def_val : Constant  Value=0
  R1_def_val : Constant  Value=0
  R2_def_val : Constant  Value=0
  force : Outport
  wires:
  R2_def_val/1 -> BCforce/4  "R2"
  R1_def_val/1 -> BCforce/3  "R1"
  L2_def_val/1 -> BCforce/2  "L2"
  L1_def_val/1 -> BCforce/1  "L1"
  BCforce/1 -> force/1  "force"

== system Demo_CarRealTime2D_cs/HostVehicle/Dynamics_UserSpecified/VI-CarRealTime/Input_Bus/Inputs/Main_Reboundstop/activity_flag ==
  BCactivity_flag : BusCreator
  L1_def_val : Constant
  L2_def_val : Constant
  R1_def_val : Constant
  R2_def_val : Constant
  activity_flag : Outport
  wires:
  R2_def_val/1 -> BCactivity_flag/4  "R2"
  R1_def_val/1 -> BCactivity_flag/3  "R1"
  L2_def_val/1 -> BCactivity_flag/2  "L2"
  L1_def_val/1 -> BCactivity_flag/1  "L1"
  BCactivity_flag/1 -> activity_flag/1  "activity_flag"

== system Demo_CarRealTime2D_cs/HostVehicle/Dynamics_UserSpecified/VI-CarRealTime/Input_Bus/Inputs/Main_Reboundstop/force ==
  BCforce : BusCreator
  L1_def_val : Constant  Value=0
  L2_def_val : Constant  Value=0
  R1_def_val : Constant  Value=0
  R2_def_val : Constant  Value=0
  force : Outport
  wires:
  R2_def_val/1 -> BCforce/4  "R2"
  R1_def_val/1 -> BCforce/3  "R1"
  L2_def_val/1 -> BCforce/2  "L2"
  L1_def_val/1 -> BCforce/1  "L1"
  BCforce/1 -> force/1  "force"

== system Demo_CarRealTime2D_cs/HostVehicle/Dynamics_UserSpecified/VI-CarRealTime/Input_Bus/Inputs/Main_Spring/activity_flag ==
  BCactivity_flag : BusCreator
  L1_def_val : Constant
  L2_def_val : Constant
  R1_def_val : Constant
  R2_def_val : Constant
  activity_flag : Outport
  wires:
  R2_def_val/1 -> BCactivity_flag/4  "R2"
  R1_def_val/1 -> BCactivity_flag/3  "R1"
  L2_def_val/1 -> BCactivity_flag/2  "L2"
  L1_def_val/1 -> BCactivity_flag/1  "L1"
  BCactivity_flag/1 -> activity_flag/1  "activity_flag"

== system Demo_CarRealTime2D_cs/HostVehicle/Dynamics_UserSpecified/VI-CarRealTime/Input_Bus/Inputs/Main_Spring/force ==
  BCforce : BusCreator
  L1_def_val : Constant  Value=0
  L2_def_val : Constant  Value=0
  R1_def_val : Constant  Value=0
  R2_def_val : Constant  Value=0
  force : Outport
  wires:
  R2_def_val/1 -> BCforce/4  "R2"
  R1_def_val/1 -> BCforce/3  "R1"
  L2_def_val/1 -> BCforce/2  "L2"
  L1_def_val/1 -> BCforce/1  "L1"
  BCforce/1 -> force/1  "force"

== system Demo_CarRealTime2D_cs/HostVehicle/Dynamics_UserSpecified/VI-CarRealTime/Input_Bus/Inputs/Mono_Element/Bumpstop_Damper ==
  BCBumpstop_Damper : BusCreator  Inputs=2
  front_def_val : Constant  Value=0
  rear_def_val : Constant  Value=0
  Bumpstop_Damper : Outport
  wires:
  rear_def_val/1 -> BCBumpstop_Damper/2  "rear"
  front_def_val/1 -> BCBumpstop_Damper/1  "front"
  BCBumpstop_Damper/1 -> Bumpstop_Damper/1  "Bumpstop_Damper"

== system Demo_CarRealTime2D_cs/HostVehicle/Dynamics_UserSpecified/VI-CarRealTime/Input_Bus/Inputs/Mono_Element/Bumpstop_Damper_activity_flag ==
  BCBumpstop_Damper_activity_flag : BusCreator  Inputs=2
  front_def_val : Constant
  rear_def_val : Constant
  Bumpstop_Damper_activity_flag : Outport
  wires:
  rear_def_val/1 -> BCBumpstop_Damper_activity_flag/2  "rear"
  front_def_val/1 -> BCBumpstop_Damper_activity_flag/1  "front"
  BCBumpstop_Damper_activity_flag/1 -> Bumpstop_Damper_activity_flag/1  "Bumpstop_Damper_activity_flag"

== system Demo_CarRealTime2D_cs/HostVehicle/Dynamics_UserSpecified/VI-CarRealTime/Input_Bus/Inputs/Mono_Element/Bumpstop_Spring ==
  BCBumpstop_Spring : BusCreator  Inputs=2
  front_def_val : Constant  Value=0
  rear_def_val : Constant  Value=0
  Bumpstop_Spring : Outport
  wires:
  rear_def_val/1 -> BCBumpstop_Spring/2  "rear"
  front_def_val/1 -> BCBumpstop_Spring/1  "front"
  BCBumpstop_Spring/1 -> Bumpstop_Spring/1  "Bumpstop_Spring"

== system Demo_CarRealTime2D_cs/HostVehicle/Dynamics_UserSpecified/VI-CarRealTime/Input_Bus/Inputs/Mono_Element/Bumpstop_Spring_activity_flag ==
  BCBumpstop_Spring_activity_flag : BusCreator  Inputs=2
  front_def_val : Constant
  rear_def_val : Constant
  Bumpstop_Spring_activity_flag : Outport
  wires:
  rear_def_val/1 -> BCBumpstop_Spring_activity_flag/2  "rear"
  front_def_val/1 -> BCBumpstop_Spring_activity_flag/1  "front"
  BCBumpstop_Spring_activity_flag/1 -> Bumpstop_Spring_activity_flag/1  "Bumpstop_Spring_activity_flag"

== system Demo_CarRealTime2D_cs/HostVehicle/Dynamics_UserSpecified/VI-CarRealTime/Input_Bus/Inputs/Mono_Element/Damper ==
  BCDamper : BusCreator  Inputs=2
  front_def_val : Constant  Value=0
  rear_def_val : Constant  Value=0
  Damper : Outport
  wires:
  rear_def_val/1 -> BCDamper/2  "rear"
  front_def_val/1 -> BCDamper/1  "front"
  BCDamper/1 -> Damper/1  "Damper"

== system Demo_CarRealTime2D_cs/HostVehicle/Dynamics_UserSpecified/VI-CarRealTime/Input_Bus/Inputs/Mono_Element/Damper_activity_flag ==
  BCDamper_activity_flag : BusCreator  Inputs=2
  front_def_val : Constant
  rear_def_val : Constant
  Damper_activity_flag : Outport
  wires:
  rear_def_val/1 -> BCDamper_activity_flag/2  "rear"
  front_def_val/1 -> BCDamper_activity_flag/1  "front"
  BCDamper_activity_flag/1 -> Damper_activity_flag/1  "Damper_activity_flag"

== system Demo_CarRealTime2D_cs/HostVehicle/Dynamics_UserSpecified/VI-CarRealTime/Input_Bus/Inputs/Mono_Element/Inerter ==
  BCInerter : BusCreator  Inputs=2
  front_def_val : Constant  Value=0
  rear_def_val : Constant  Value=0
  Inerter : Outport
  wires:
  rear_def_val/1 -> BCInerter/2  "rear"
  front_def_val/1 -> BCInerter/1  "front"
  BCInerter/1 -> Inerter/1  "Inerter"

== system Demo_CarRealTime2D_cs/HostVehicle/Dynamics_UserSpecified/VI-CarRealTime/Input_Bus/Inputs/Mono_Element/Inerter_activity_flag ==
  BCInerter_activity_flag : BusCreator  Inputs=2
  front_def_val : Constant
  rear_def_val : Constant
  Inerter_activity_flag : Outport
  wires:
  rear_def_val/1 -> BCInerter_activity_flag/2  "rear"
  front_def_val/1 -> BCInerter_activity_flag/1  "front"
  BCInerter_activity_flag/1 -> Inerter_activity_flag/1  "Inerter_activity_flag"

== system Demo_CarRealTime2D_cs/HostVehicle/Dynamics_UserSpecified/VI-CarRealTime/Input_Bus/Inputs/Mono_Element/Reboundstop_Damper ==
  BCReboundstop_Damper : BusCreator  Inputs=2
  front_def_val : Constant  Value=0
  rear_def_val : Constant  Value=0
  Reboundstop_Damper : Outport
  wires:
  rear_def_val/1 -> BCReboundstop_Damper/2  "rear"
  front_def_val/1 -> BCReboundstop_Damper/1  "front"
  BCReboundstop_Damper/1 -> Reboundstop_Damper/1  "Reboundstop_Damper"

== system Demo_CarRealTime2D_cs/HostVehicle/Dynamics_UserSpecified/VI-CarRealTime/Input_Bus/Inputs/Mono_Element/Reboundstop_Damper_activity_flag ==
  BCReboundstop_Damper_activity_flag : BusCreator  Inputs=2
  front_def_val : Constant
  rear_def_val : Constant
  Reboundstop_Damper_activity_flag : Outport
  wires:
  rear_def_val/1 -> BCReboundstop_Damper_activity_flag/2  "rear"
  front_def_val/1 -> BCReboundstop_Damper_activity_flag/1  "front"
  BCReboundstop_Damper_activity_flag/1 -> Reboundstop_Damper_activity_flag/1  "Reboundstop_Damper_activity_flag"
